simulink model "simulinkk"  (R2016b)
settings: Solver=VariableStepAuto  StartTime=0.0  StopTime=10  RelTol=1e-3
undefined symbols (not defined in the file): AA, BB, C, CC, K, L
settings Model: Creator=apple  LastModifiedBy=apple
settings SimMechanicsCC: VisOnUpdateDiagram=on  VisDuringSimulation=on

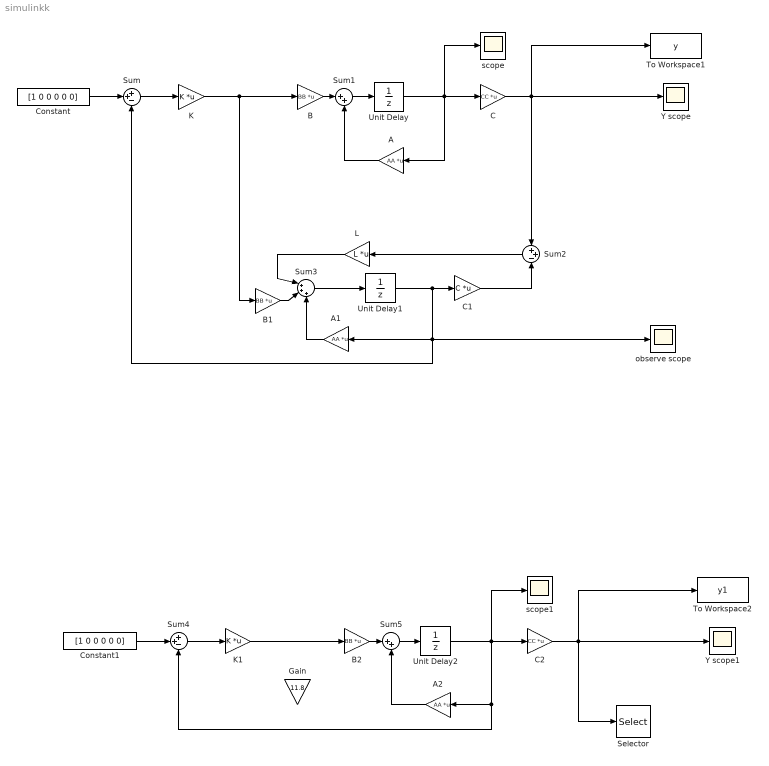
== system simulinkk ==
  A : Gain  Gain=AA  Multiplication=Matrix(K*u)
  A1 : Gain  Gain=AA  Multiplication=Matrix(K*u)
  A2 : Gain  Gain=AA  Multiplication=Matrix(K*u)
  B : Gain  Gain=BB  Multiplication=Matrix(K*u)
  B1 : Gain  Gain=BB  Multiplication=Matrix(K*u)
  B2 : Gain  Gain=BB  Multiplication=Matrix(K*u)
  C : Gain  Gain=CC  Multiplication=Matrix(K*u)
  C1 : Gain  Gain=C  Multiplication=Matrix(K*u)
  C2 : Gain  Gain=CC  Multiplication=Matrix(K*u)
  Constant : Constant  Value=[1 0 0 0 0 0]
  Constant1 : Constant  Value=[1 0 0 0 0 0]
  Gain : Gain  Gain=11.8
  K : Gain  Gain=K  Multiplication=Matrix(K*u)
  K1 : Gain  Gain=K  Multiplication=Matrix(K*u)
  L : Gain  Gain=L  Multiplication=Matrix(K*u)
  Selector : Selector  InputPortWidth=3  IndexOptions=Index vector (dialog)  Indices=[1 ]  OutputSizes=1
  Sum : Sum  Inputs=++-
  Sum1 : Sum  Inputs=|++
  Sum2 : Sum  Inputs=++-
  Sum3 : Sum  Inputs=|+++
  Sum4 : Sum  Inputs=++-
  Sum5 : Sum  Inputs=|++
  To Workspace1 : ToWorkspace  VariableName=y  SaveFormat=Timeseries  SampleTime=-1
  To Workspace2 : ToWorkspace  VariableName=y1  SaveFormat=Timeseries  SampleTime=-1
  Unit Delay : UnitDelay  SampleTime=0.01
  Unit Delay1 : UnitDelay  SampleTime=0.01
  Unit Delay2 : UnitDelay  SampleTime=0.01
  Y scope : Scope
  Y scope1 : Scope
  observe scope : Scope
  scope : Scope
  scope1 : Scope
  wires:
  Sum1/1 -> Unit Delay/1
  B/1 -> Sum1/1
  A/1 -> Sum1/2
  C/1 -> Sum2/1, Y scope/1, To Workspace1/1
  Unit Delay/1 -> A/1, C/1, scope/1
  Sum2/1 -> L/1
  Sum3/1 -> Unit Delay1/1
  C1/1 -> Sum2/3
  B1/1 -> Sum3/2
  A1/1 -> Sum3/3
  L/1 -> Sum3/1
  K/1 -> B1/1, B/1
  Constant/1 -> Sum/2
  Sum/1 -> K/1
  Unit Delay1/1 -> Sum/3, A1/1, observe scope/1, C1/1
  Sum5/1 -> Unit Delay2/1
  B2/1 -> Sum5/1
  A2/1 -> Sum5/2
  C2/1 -> Selector/1, Y scope1/1, To Workspace2/1
  Unit Delay2/1 -> Sum4/3, A2/1, C2/1, scope1/1
  K1/1 -> B2/1
  Constant1/1 -> Sum4/2
  Sum4/1 -> K1/1
